simulink model "DoubleJoints_Algorithm"  (R2018b)
settings: Solver=FixedStepDiscrete  StartTime=0.0  StopTime=Inf  FixedStep=0.001  RelTol=1e-3  EnableMultiTasking=on
undefined symbols (not defined in the file): J2, J7, Motor_Current, Motor_Position, Motor_Velocity, Send_GUIdata
libraries: c280xlib x20, simulink x9, dspsrcs4 x2, idelinklib_common x1
(part 2 of 3)

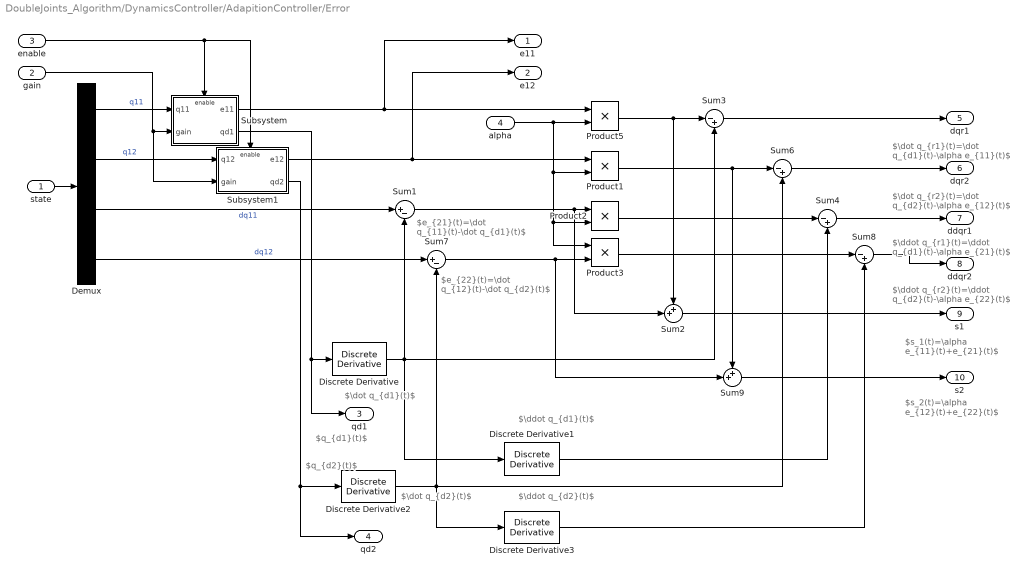
== system DoubleJoints_Algorithm/DynamicsController/AdapitionController/Error  ==
  note: $\dot q_{r2}(t)=\dot q_{d2}(t)-\alpha e_{12}(t)$
  note: $\dot q_{r1}(t)=\dot q_{d1}(t)-\alpha e_{11}(t)$
  note: $\ddot q_{r1}(t)=\ddot q_{d1}(t)-\alpha e_{21}(t)$
  note: $\ddot q_{r2}(t)=\ddot q_{d2}(t)-\alpha e_{22}(t)$
  note: $s_1(t)=\alpha e_{11}(t)+e_{21}(t)$
  note: $s_2(t)=\alpha e_{12}(t)+e_{22}(t)$
  note: $e_{21}(t)=\dot q_{11}(t)-\dot q_{d1}(t)$
  note: $e_{22}(t)=\dot q_{12}(t)-\dot q_{d2}(t)$
  note: $\dot q_{d2}(t)$
  note: $\dot q_{d1}(t)$
  note: $\ddot q_{d1}(t)$
  note: $q_{d1}(t)$
  note: $\ddot q_{d2}(t)$
  note: $q_{d2}(t)$
  state : Inport
  gain : Inport  Port=2
  enable : Inport  Port=3
  alpha : Inport  Port=4
  Demux : Demux
  Discrete Derivative{,1..3} (4 alike) : simulink/Discrete/Discrete Derivative  gainval=1.0  ICPrevScaledInput=0.0  OutMin=[]  OutMax=[]  OutDataType=fixdt(1, 16)  OutScaling=2^-10  DoSatur=off
  Product{1..3,5} (4 alike) : Product
  Subsystem : Subsystem  Priority=1
      settings: RTWSystemCode=Nonreusable function
  Subsystem1 : Subsystem  Priority=2
      settings: RTWSystemCode=Nonreusable function
  Sum1 : Sum  Inputs=|+-
  Sum2 : Sum  Inputs=++|
  Sum{3..4,6,8} (4 alike) : Sum  Inputs=|-+
  Sum7 : Sum  Inputs=|+-
  Sum9 : Sum  Inputs=++|
  e11 : Outport
  e12 : Outport  Port=2
  qd1 : Outport  Port=3
  qd2 : Outport  Port=4
  dqr1 : Outport  Port=5
  dqr2 : Outport  Port=6
  ddqr1 : Outport  Port=7
  ddqr2 : Outport  Port=8
  s1 : Outport  Port=9
  s2 : Outport  Port=10
  wires:
  state/1 -> Demux/1
  Demux/1 -> Subsystem/1(q11)  "q11"
  Demux/3 -> Sum1/1  "dq11"
  Subsystem/2(qd1) -> Discrete Derivative/1, qd1/1
  Product5/1 -> Sum3/1, Sum2/1
  Sum3/1 -> dqr1/1
  Sum1/1 -> Product2/1, Sum2/2
  Product2/1 -> Sum4/1
  Discrete Derivative/1 -> Sum3/2, Discrete Derivative1/1, Sum1/2
  Sum4/1 -> ddqr1/1
  Sum2/1 -> s1/1
  Demux/2 -> Subsystem1/1(q12)  "q12"
  Product1/1 -> Sum6/1, Sum9/1
  Sum6/1 -> dqr2/1
  Demux/4 -> Sum7/1  "dq12"
  Sum7/1 -> Sum9/2, Product3/2
  Product3/1 -> Sum8/1
  Subsystem1/2(qd2) -> qd2/1, Discrete Derivative2/1
  Sum8/1 -> ddqr2/1
  Sum9/1 -> s2/1
  alpha/1 -> Product5/2, Product1/2, Product2/2, Product3/1
  Discrete Derivative1/1 -> Sum4/2
  Discrete Derivative3/1 -> Sum8/2
  Discrete Derivative2/1 -> Discrete Derivative3/1, Sum6/2, Sum7/2
  enable/1 -> Subsystem/Enable, Subsystem1/Enable
  Subsystem/1(e11) -> e11/1, Product5/1
  Subsystem1/1(e12) -> e12/1, Product1/1
  gain/1 -> Subsystem1/2(gain), Subsystem/2(gain)

== system DoubleJoints_Algorithm/DynamicsController/DriverTwoMotor/BottomDriver ==
  SelectJoint1 : Inport
  SelectJoint2 : Inport  Port=2
  MSG1 : Inport  Port=3
  MSG2 : Inport  Port=4
  Enable : EnablePort
  Judgement : Subsystem
  Relational Operator : RelationalOperator  Operator=~=  OutDataTypeStr=boolean  RndMeth=Simplest
  wires:
  MSG1/1 -> Judgement/3(MSG1)
  MSG2/1 -> Judgement/4(MSG2)
  SelectJoint1/1 -> Judgement/1(SelectJointOne), Relational Operator/1
  SelectJoint2/1 -> Judgement/2(SelectJointTwo), Relational Operator/2
  Relational Operator/1 -> Judgement/Enable

== system DoubleJoints_Algorithm/DynamicsController/DriverTwoMotor/驱动器指令 ==
  Current1 : Inport
  Current2 : Inport  Port=2
  enable : Inport  Port=3
  Chart2 : Stateflow chart  TreatAsAtomicUnit=on
  Data Store Read : DataStoreRead  DataStoreName=StartRobot
  Data Type Conversion1 : DataTypeConversion  OutDataTypeStr=uint8
  Data Type Conversion2 : DataTypeConversion  OutDataTypeStr=uint16
  Data Type Conversion3 : DataTypeConversion  OutDataTypeStr=uint8
  Data Type Conversion4 : DataTypeConversion  OutDataTypeStr=uint16
  Data Type Conversion7 : DataTypeConversion  OutDataTypeStr=uint16
  MSG1 : Outport
  MSG2 : Outport  Port=2
  wires:
  Data Type Conversion1/1 -> MSG1/1
  Chart2/1(MSG1) -> Data Type Conversion1/1
  Current2/1 -> Data Type Conversion7/1
  Data Type Conversion7/1 -> Chart2/2(Current2)
  Current1/1 -> Data Type Conversion2/1
  Data Type Conversion2/1 -> Chart2/1(Current1)
  Data Type Conversion3/1 -> MSG2/1
  Chart2/2(MSG2) -> Data Type Conversion3/1
  Data Type Conversion4/1 -> Chart2/3(write)
  enable/1 -> Data Type Conversion4/1
  Data Store Read/1 -> Chart2/4(StartRobot)

== system DoubleJoints_Algorithm/DynamicsController/GetAngle1/Joint1 ==
  note: 内转子位置的脉冲值
  Action Port : ActionPort
  Data Store Read5 : DataStoreRead  DataStoreName=Motor_Position  DataStoreElements=Motor_Position(1)
  Joint1 : Outport
  wires:
  Data Store Read5/1 -> Joint1/1

== system DoubleJoints_Algorithm/DynamicsController/GetAngle1/Joint2 ==
  Action Port : ActionPort
  Data Store Read5 : DataStoreRead  DataStoreName=Motor_Position  DataStoreElements=Motor_Position(2)
  Joint2 : Outport
  wires:
  Data Store Read5/1 -> Joint2/1

== system DoubleJoints_Algorithm/DynamicsController/GetAngle1/Joint3 ==
  Action Port : ActionPort
  Data Store Read5 : DataStoreRead  DataStoreName=Motor_Position  DataStoreElements=Motor_Position(3)
  Joint3 : Outport
  wires:
  Data Store Read5/1 -> Joint3/1

== system DoubleJoints_Algorithm/DynamicsController/GetAngle1/Joint4 ==
  Action Port : ActionPort
  Data Store Read5 : DataStoreRead  DataStoreName=Motor_Position  DataStoreElements=Motor_Position(4)
  Joint4 : Outport
  wires:
  Data Store Read5/1 -> Joint4/1

== system DoubleJoints_Algorithm/DynamicsController/GetAngle1/Joint5 ==
  Action Port : ActionPort
  Data Store Read5 : DataStoreRead  DataStoreName=Motor_Position  DataStoreElements=Motor_Position(5)
  Joint5 : Outport
  wires:
  Data Store Read5/1 -> Joint5/1

== system DoubleJoints_Algorithm/DynamicsController/GetAngle1/Joint6 ==
  Action Port : ActionPort
  Data Store Read5 : DataStoreRead  DataStoreName=Motor_Position  DataStoreElements=Motor_Position(6)
  Joint6 : Outport
  wires:
  Data Store Read5/1 -> Joint6/1

== system DoubleJoints_Algorithm/DynamicsController/GetAngle2/Joint1 ==
  note: 内转子位置的脉冲值
  Action Port : ActionPort
  Data Store Read5 : DataStoreRead  DataStoreName=Motor_Position  DataStoreElements=Motor_Position(1)
  Joint1 : Outport
  wires:
  Data Store Read5/1 -> Joint1/1

== system DoubleJoints_Algorithm/DynamicsController/GetAngle2/Joint2 ==
  Action Port : ActionPort
  Data Store Read5 : DataStoreRead  DataStoreName=Motor_Position  DataStoreElements=Motor_Position(2)
  Joint2 : Outport
  wires:
  Data Store Read5/1 -> Joint2/1

== system DoubleJoints_Algorithm/DynamicsController/GetAngle2/Joint3 ==
  Action Port : ActionPort
  Data Store Read5 : DataStoreRead  DataStoreName=Motor_Position  DataStoreElements=Motor_Position(3)
  Joint3 : Outport
  wires:
  Data Store Read5/1 -> Joint3/1

== system DoubleJoints_Algorithm/DynamicsController/GetAngle2/Joint4 ==
  Action Port : ActionPort
  Data Store Read5 : DataStoreRead  DataStoreName=Motor_Position  DataStoreElements=Motor_Position(4)
  Joint4 : Outport
  wires:
  Data Store Read5/1 -> Joint4/1

== system DoubleJoints_Algorithm/DynamicsController/GetAngle2/Joint5 ==
  Action Port : ActionPort
  Data Store Read5 : DataStoreRead  DataStoreName=Motor_Position  DataStoreElements=Motor_Position(5)
  Joint5 : Outport
  wires:
  Data Store Read5/1 -> Joint5/1

== system DoubleJoints_Algorithm/DynamicsController/GetAngle2/Joint6 ==
  Action Port : ActionPort
  Data Store Read5 : DataStoreRead  DataStoreName=Motor_Position  DataStoreElements=Motor_Position(6)
  Joint6 : Outport
  wires:
  Data Store Read5/1 -> Joint6/1

== system DoubleJoints_Algorithm/DynamicsController/GetAngleSpeed/Joint1 ==
  note: 内转子速度
      | 的脉冲值
  Action Port : ActionPort  ActionType=case
  Data Store Read1 : DataStoreRead  DataStoreName=Motor_Velocity  DataStoreElements=Motor_Velocity(1)
  Joint1_Velocity : Outport
  wires:
  Data Store Read1/1 -> Joint1_Velocity/1

== system DoubleJoints_Algorithm/DynamicsController/GetAngleSpeed/Joint2 ==
  note: 内转子速度
      | 的脉冲值
  Action Port : ActionPort  ActionType=case
  Data Store Read1 : DataStoreRead  DataStoreName=Motor_Velocity  DataStoreElements=Motor_Velocity(2)
  Joint2_Velocity : Outport
  wires:
  Data Store Read1/1 -> Joint2_Velocity/1

== system DoubleJoints_Algorithm/DynamicsController/GetAngleSpeed/Joint3 ==
  note: 内转子速度
      | 的脉冲值
  Action Port : ActionPort  ActionType=case
  Data Store Read1 : DataStoreRead  DataStoreName=Motor_Velocity  DataStoreElements=Motor_Velocity(3)
  Joint3_Velocity : Outport
  wires:
  Data Store Read1/1 -> Joint3_Velocity/1

== system DoubleJoints_Algorithm/DynamicsController/GetAngleSpeed/Joint4 ==
  note: 内转子速度
      | 的脉冲值
  Action Port : ActionPort  ActionType=case
  Data Store Read1 : DataStoreRead  DataStoreName=Motor_Velocity  DataStoreElements=Motor_Velocity(4)
  Joint4_Velocity : Outport
  wires:
  Data Store Read1/1 -> Joint4_Velocity/1

== system DoubleJoints_Algorithm/DynamicsController/GetAngleSpeed/Joint5 ==
  note: 内转子速度
      | 的脉冲值
  Action Port : ActionPort  ActionType=case
  Data Store Read1 : DataStoreRead  DataStoreName=Motor_Velocity  DataStoreElements=Motor_Velocity(5)
  Joint5_Velocity : Outport
  wires:
  Data Store Read1/1 -> Joint5_Velocity/1

== system DoubleJoints_Algorithm/DynamicsController/GetAngleSpeed/Joint6 ==
  note: 内转子速度
      | 的脉冲值
  Action Port : ActionPort  ActionType=case
  Data Store Read1 : DataStoreRead  DataStoreName=Motor_Velocity  DataStoreElements=Motor_Velocity(6)
  Joint6_Velocity : Outport
  wires:
  Data Store Read1/1 -> Joint6_Velocity/1

== system DoubleJoints_Algorithm/DynamicsController/GetAngleSpeed1/Joint1 ==
  note: 内转子速度
      | 的脉冲值
  Action Port : ActionPort  ActionType=case
  Data Store Read1 : DataStoreRead  DataStoreName=Motor_Velocity  DataStoreElements=Motor_Velocity(1)
  Joint1_Velocity : Outport
  wires:
  Data Store Read1/1 -> Joint1_Velocity/1

== system DoubleJoints_Algorithm/DynamicsController/GetAngleSpeed1/Joint2 ==
  note: 内转子速度
      | 的脉冲值
  Action Port : ActionPort  ActionType=case
  Data Store Read1 : DataStoreRead  DataStoreName=Motor_Velocity  DataStoreElements=Motor_Velocity(2)
  Joint2_Velocity : Outport
  wires:
  Data Store Read1/1 -> Joint2_Velocity/1

== system DoubleJoints_Algorithm/DynamicsController/GetAngleSpeed1/Joint3 ==
  note: 内转子速度
      | 的脉冲值
  Action Port : ActionPort  ActionType=case
  Data Store Read1 : DataStoreRead  DataStoreName=Motor_Velocity  DataStoreElements=Motor_Velocity(3)
  Joint3_Velocity : Outport
  wires:
  Data Store Read1/1 -> Joint3_Velocity/1

== system DoubleJoints_Algorithm/DynamicsController/GetAngleSpeed1/Joint4 ==
  note: 内转子速度
      | 的脉冲值
  Action Port : ActionPort  ActionType=case
  Data Store Read1 : DataStoreRead  DataStoreName=Motor_Velocity  DataStoreElements=Motor_Velocity(4)
  Joint4_Velocity : Outport
  wires:
  Data Store Read1/1 -> Joint4_Velocity/1

== system DoubleJoints_Algorithm/DynamicsController/GetAngleSpeed1/Joint5 ==
  note: 内转子速度
      | 的脉冲值
  Action Port : ActionPort  ActionType=case
  Data Store Read1 : DataStoreRead  DataStoreName=Motor_Velocity  DataStoreElements=Motor_Velocity(5)
  Joint5_Velocity : Outport
  wires:
  Data Store Read1/1 -> Joint5_Velocity/1

== system DoubleJoints_Algorithm/DynamicsController/GetAngleSpeed1/Joint6 ==
  note: 内转子速度
      | 的脉冲值
  Action Port : ActionPort  ActionType=case
  Data Store Read1 : DataStoreRead  DataStoreName=Motor_Velocity  DataStoreElements=Motor_Velocity(6)
  Joint6_Velocity : Outport
  wires:
  Data Store Read1/1 -> Joint6_Velocity/1

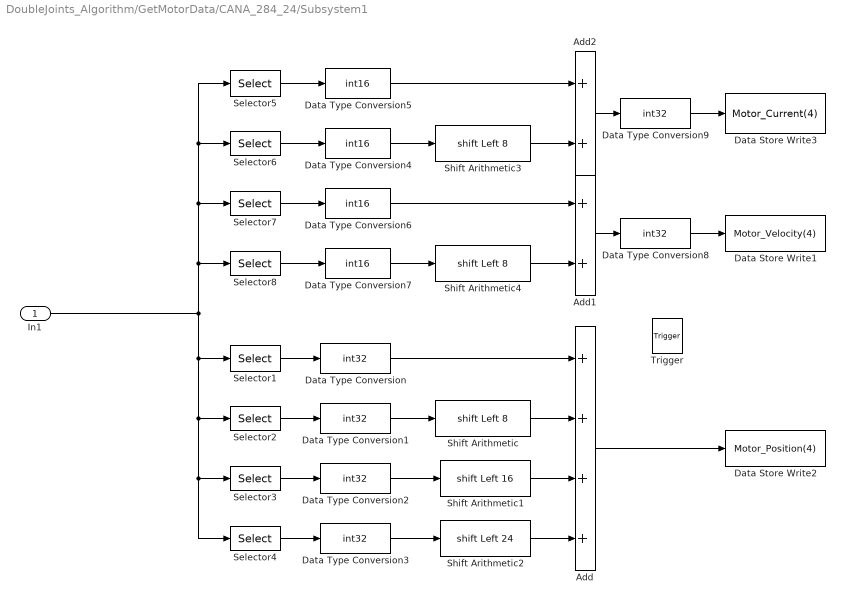
== system DoubleJoints_Algorithm/GetMotorData/CANA_284_24/Subsystem1 ==
  In1 : Inport
  Trigger : TriggerPort  TriggerType=function-call  VariantControl=Variant  PortDimensions=1
  Add : Sum  Inputs=4
  Add1 : Sum  Inputs=2
  Add2 : Sum  Inputs=2
  Data Store Write1 : DataStoreWrite  DataStoreName=Motor_Velocity  DataStoreElements=Motor_Velocity(4)
  Data Store Write2 : DataStoreWrite  DataStoreName=Motor_Position  DataStoreElements=Motor_Position(4)
  Data Store Write3 : DataStoreWrite  DataStoreName=Motor_Current  DataStoreElements=Motor_Current(4)
  Data Type Conversion{,1..3,8..9} (6 alike) : DataTypeConversion  OutDataTypeStr=int32
  Data Type Conversion{4..7} (4 alike) : DataTypeConversion  OutDataTypeStr=int16
  Selector1 : Selector  IndexMode=Zero-based  InputPortWidth=8  IndexOptions=Index vector (dialog)  Indices=4  OutputSizes=1
  Selector2 : Selector  IndexMode=Zero-based  InputPortWidth=8  IndexOptions=Index vector (dialog)  Indices=5  OutputSizes=1
  Selector3 : Selector  IndexMode=Zero-based  InputPortWidth=8  IndexOptions=Index vector (dialog)  Indices=6  OutputSizes=1
  Selector4 : Selector  IndexMode=Zero-based  InputPortWidth=8  IndexOptions=Index vector (dialog)  Indices=7  OutputSizes=1
  Selector5 : Selector  IndexMode=Zero-based  InputPortWidth=8  IndexOptions=Index vector (dialog)  Indices=0  OutputSizes=1
  Selector6 : Selector  IndexMode=Zero-based  InputPortWidth=8  IndexOptions=Index vector (dialog)  Indices=1  OutputSizes=1
  Selector7 : Selector  IndexMode=Zero-based  InputPortWidth=8  IndexOptions=Index vector (dialog)  Indices=2  OutputSizes=1
  Selector8 : Selector  IndexMode=Zero-based  InputPortWidth=8  IndexOptions=Index vector (dialog)  Indices=3  OutputSizes=1
  Shift Arithmetic : ArithShift  BitShiftNumber=8  BitShiftDirection=Left
  Shift Arithmetic1 : ArithShift  BitShiftNumber=16  BitShiftDirection=Left
  Shift Arithmetic2 : ArithShift  BitShiftNumber=24  BitShiftDirection=Left
  Shift Arithmetic3 : ArithShift  BitShiftNumber=8  BitShiftDirection=Left
  Shift Arithmetic4 : ArithShift  BitShiftNumber=8  BitShiftDirection=Left
  wires:
  Selector3/1 -> Data Type Conversion2/1
  Shift Arithmetic/1 -> Add/2
  Shift Arithmetic2/1 -> Add/4
  Data Type Conversion/1 -> Add/1
  Selector1/1 -> Data Type Conversion/1
  Selector4/1 -> Data Type Conversion3/1
  Add/1 -> Data Store Write2/1
  Shift Arithmetic1/1 -> Add/3
  Selector2/1 -> Data Type Conversion1/1
  Data Type Conversion7/1 -> Shift Arithmetic4/1
  Data Type Conversion6/1 -> Add1/1
  Selector7/1 -> Data Type Conversion6/1
  Selector8/1 -> Data Type Conversion7/1
  Selector6/1 -> Data Type Conversion4/1
  In1/1 -> Selector3/1, Selector4/1, Selector2/1, Selector1/1, Selector5/1, Selector6/1, Selector7/1, Selector8/1
  Add1/1 -> Data Type Conversion8/1
  Shift Arithmetic4/1 -> Add1/2
  Data Type Conversion1/1 -> Shift Arithmetic/1
  Data Type Conversion2/1 -> Shift Arithmetic1/1
  Data Type Conversion3/1 -> Shift Arithmetic2/1
  Selector5/1 -> Data Type Conversion5/1
  Data Type Conversion4/1 -> Shift Arithmetic3/1
  Data Type Conversion8/1 -> Data Store Write1/1
  Shift Arithmetic3/1 -> Add2/2
  Data Type Conversion5/1 -> Add2/1
  Add2/1 -> Data Type Conversion9/1
  Data Type Conversion9/1 -> Data Store Write3/1

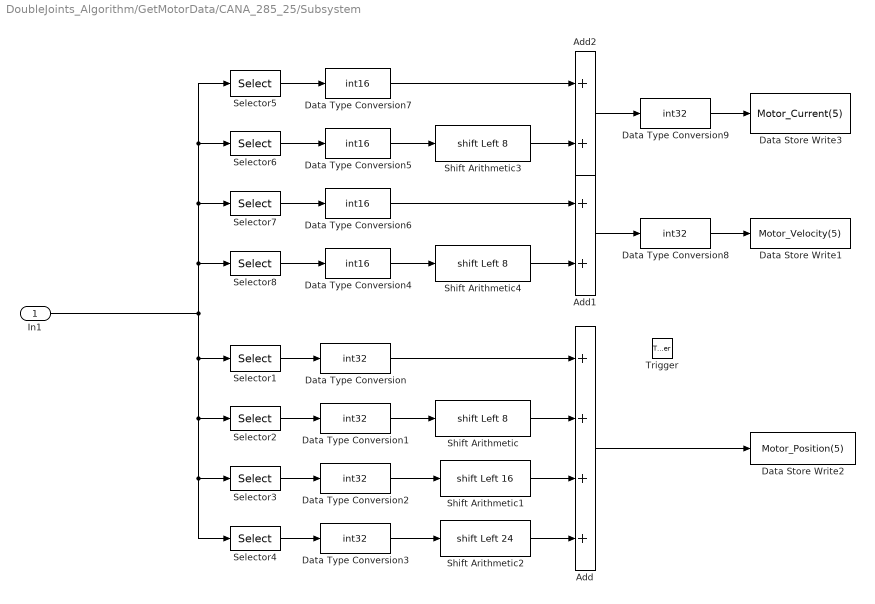
== system DoubleJoints_Algorithm/GetMotorData/CANA_285_25/Subsystem ==
  In1 : Inport
  Trigger : TriggerPort  TriggerType=function-call  VariantControl=Variant  PortDimensions=1
  Add : Sum  Inputs=4
  Add1 : Sum  Inputs=2
  Add2 : Sum  Inputs=2
  Data Store Write1 : DataStoreWrite  DataStoreName=Motor_Velocity  DataStoreElements=Motor_Velocity(5)
  Data Store Write2 : DataStoreWrite  DataStoreName=Motor_Position  DataStoreElements=Motor_Position(5)
  Data Store Write3 : DataStoreWrite  DataStoreName=Motor_Current  DataStoreElements=Motor_Current(5)
  Data Type Conversion{,1..3,8..9} (6 alike) : DataTypeConversion  OutDataTypeStr=int32
  Data Type Conversion{4..7} (4 alike) : DataTypeConversion  OutDataTypeStr=int16
  Selector1 : Selector  IndexMode=Zero-based  InputPortWidth=8  IndexOptions=Index vector (dialog)  Indices=4  OutputSizes=1
  Selector2 : Selector  IndexMode=Zero-based  InputPortWidth=8  IndexOptions=Index vector (dialog)  Indices=5  OutputSizes=1
  Selector3 : Selector  IndexMode=Zero-based  InputPortWidth=8  IndexOptions=Index vector (dialog)  Indices=6  OutputSizes=1
  Selector4 : Selector  IndexMode=Zero-based  InputPortWidth=8  IndexOptions=Index vector (dialog)  Indices=7  OutputSizes=1
  Selector5 : Selector  IndexMode=Zero-based  InputPortWidth=8  IndexOptions=Index vector (dialog)  Indices=0  OutputSizes=1
  Selector6 : Selector  IndexMode=Zero-based  InputPortWidth=8  IndexOptions=Index vector (dialog)  Indices=1  OutputSizes=1
  Selector7 : Selector  IndexMode=Zero-based  InputPortWidth=8  IndexOptions=Index vector (dialog)  Indices=2  OutputSizes=1
  Selector8 : Selector  IndexMode=Zero-based  InputPortWidth=8  IndexOptions=Index vector (dialog)  Indices=3  OutputSizes=1
  Shift Arithmetic : ArithShift  BitShiftNumber=8  BitShiftDirection=Left
  Shift Arithmetic1 : ArithShift  BitShiftNumber=16  BitShiftDirection=Left
  Shift Arithmetic2 : ArithShift  BitShiftNumber=24  BitShiftDirection=Left
  Shift Arithmetic3 : ArithShift  BitShiftNumber=8  BitShiftDirection=Left
  Shift Arithmetic4 : ArithShift  BitShiftNumber=8  BitShiftDirection=Left
  wires:
  Selector3/1 -> Data Type Conversion2/1
  Shift Arithmetic/1 -> Add/2
  Shift Arithmetic2/1 -> Add/4
  Data Type Conversion/1 -> Add/1
  Selector1/1 -> Data Type Conversion/1
  Selector4/1 -> Data Type Conversion3/1
  Add/1 -> Data Store Write2/1
  Shift Arithmetic1/1 -> Add/3
  Selector2/1 -> Data Type Conversion1/1
  Selector5/1 -> Data Type Conversion7/1
  Selector8/1 -> Data Type Conversion4/1
  Data Type Conversion4/1 -> Shift Arithmetic4/1
  Data Type Conversion6/1 -> Add1/1
  Selector7/1 -> Data Type Conversion6/1
  Selector6/1 -> Data Type Conversion5/1
  In1/1 -> Selector3/1, Selector4/1, Selector2/1, Selector1/1, Selector5/1, Selector6/1, Selector7/1, Selector8/1
  Add1/1 -> Data Type Conversion8/1
  Data Type Conversion1/1 -> Shift Arithmetic/1
  Data Type Conversion2/1 -> Shift Arithmetic1/1
  Data Type Conversion3/1 -> Shift Arithmetic2/1
  Data Type Conversion5/1 -> Shift Arithmetic3/1
  Shift Arithmetic4/1 -> Add1/2
  Shift Arithmetic3/1 -> Add2/2
  Data Type Conversion7/1 -> Add2/1
  Add2/1 -> Data Type Conversion9/1
  Data Type Conversion8/1 -> Data Store Write1/1
  Data Type Conversion9/1 -> Data Store Write3/1

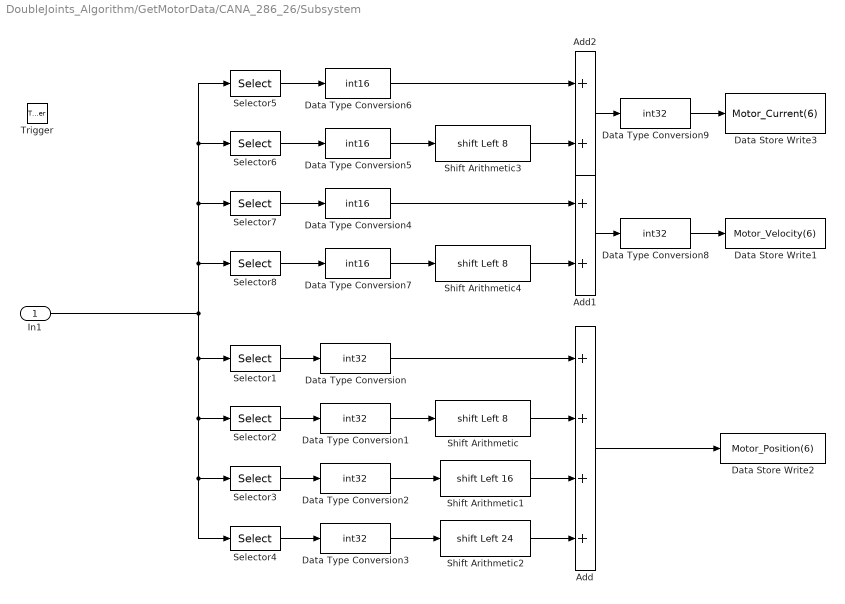
== system DoubleJoints_Algorithm/GetMotorData/CANA_286_26/Subsystem ==
  In1 : Inport
  Trigger : TriggerPort  TriggerType=function-call  VariantControl=Variant  PortDimensions=1
  Add : Sum  Inputs=4
  Add1 : Sum  Inputs=2
  Add2 : Sum  Inputs=2
  Data Store Write1 : DataStoreWrite  DataStoreName=Motor_Velocity  DataStoreElements=Motor_Velocity(6)
  Data Store Write2 : DataStoreWrite  DataStoreName=Motor_Position  DataStoreElements=Motor_Position(6)
  Data Store Write3 : DataStoreWrite  DataStoreName=Motor_Current  DataStoreElements=Motor_Current(6)
  Data Type Conversion{,1..3,8..9} (6 alike) : DataTypeConversion  OutDataTypeStr=int32
  Data Type Conversion{4..7} (4 alike) : DataTypeConversion  OutDataTypeStr=int16
  Selector1 : Selector  IndexMode=Zero-based  InputPortWidth=8  IndexOptions=Index vector (dialog)  Indices=4  OutputSizes=1
  Selector2 : Selector  IndexMode=Zero-based  InputPortWidth=8  IndexOptions=Index vector (dialog)  Indices=5  OutputSizes=1
  Selector3 : Selector  IndexMode=Zero-based  InputPortWidth=8  IndexOptions=Index vector (dialog)  Indices=6  OutputSizes=1
  Selector4 : Selector  IndexMode=Zero-based  InputPortWidth=8  IndexOptions=Index vector (dialog)  Indices=7  OutputSizes=1
  Selector5 : Selector  IndexMode=Zero-based  InputPortWidth=8  IndexOptions=Index vector (dialog)  Indices=0  OutputSizes=1
  Selector6 : Selector  IndexMode=Zero-based  InputPortWidth=8  IndexOptions=Index vector (dialog)  Indices=1  OutputSizes=1
  Selector7 : Selector  IndexMode=Zero-based  InputPortWidth=8  IndexOptions=Index vector (dialog)  Indices=2  OutputSizes=1
  Selector8 : Selector  IndexMode=Zero-based  InputPortWidth=8  IndexOptions=Index vector (dialog)  Indices=3  OutputSizes=1
  Shift Arithmetic : ArithShift  BitShiftNumber=8  BitShiftDirection=Left
  Shift Arithmetic1 : ArithShift  BitShiftNumber=16  BitShiftDirection=Left
  Shift Arithmetic2 : ArithShift  BitShiftNumber=24  BitShiftDirection=Left
  Shift Arithmetic3 : ArithShift  BitShiftNumber=8  BitShiftDirection=Left
  Shift Arithmetic4 : ArithShift  BitShiftNumber=8  BitShiftDirection=Left
  wires:
  Selector3/1 -> Data Type Conversion2/1
  Shift Arithmetic/1 -> Add/2
  Shift Arithmetic2/1 -> Add/4
  Data Type Conversion/1 -> Add/1
  Selector1/1 -> Data Type Conversion/1
  Selector4/1 -> Data Type Conversion3/1
  Add/1 -> Data Store Write2/1
  Shift Arithmetic1/1 -> Add/3
  Selector2/1 -> Data Type Conversion1/1
  Selector5/1 -> Data Type Conversion6/1
  Data Type Conversion7/1 -> Shift Arithmetic4/1
  Selector7/1 -> Data Type Conversion4/1
  Selector8/1 -> Data Type Conversion7/1
  Selector6/1 -> Data Type Conversion5/1
  In1/1 -> Selector3/1, Selector4/1, Selector2/1, Selector1/1, Selector5/1, Selector6/1, Selector7/1, Selector8/1
  Add1/1 -> Data Type Conversion8/1
  Data Type Conversion1/1 -> Shift Arithmetic/1
  Data Type Conversion2/1 -> Shift Arithmetic1/1
  Data Type Conversion3/1 -> Shift Arithmetic2/1
  Shift Arithmetic4/1 -> Add1/2
  Data Type Conversion4/1 -> Add1/1
  Data Type Conversion5/1 -> Shift Arithmetic3/1
  Data Type Conversion6/1 -> Add2/1
  Shift Arithmetic3/1 -> Add2/2
  Add2/1 -> Data Type Conversion9/1
  Data Type Conversion8/1 -> Data Store Write1/1
  Data Type Conversion9/1 -> Data Store Write3/1

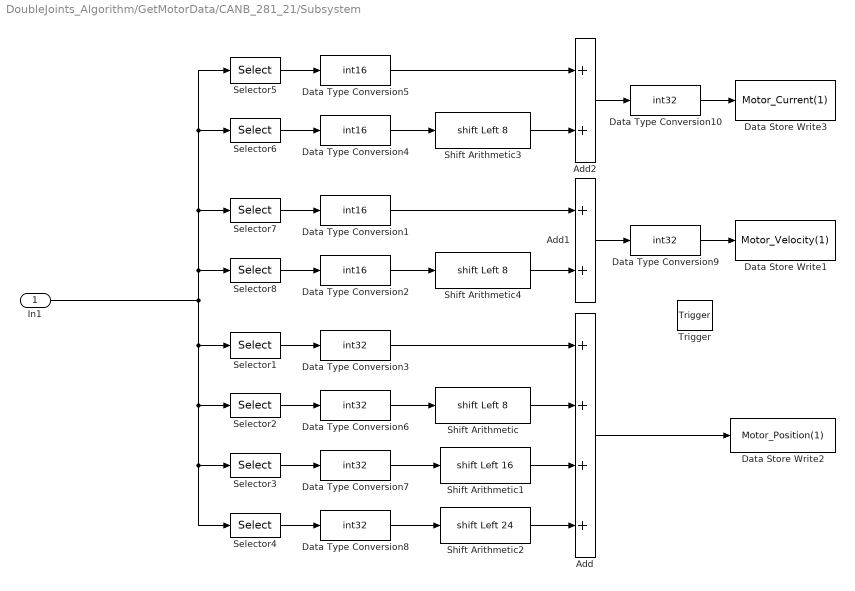
== system DoubleJoints_Algorithm/GetMotorData/CANB_281_21/Subsystem ==
  In1 : Inport
  Trigger : TriggerPort  TriggerType=function-call  VariantControl=Variant  PortDimensions=1
  Add : Sum  Inputs=4
  Add1 : Sum  Inputs=2
  Add2 : Sum  Inputs=2
  Data Store Write1 : DataStoreWrite  DataStoreName=Motor_Velocity  DataStoreElements=Motor_Velocity(1)
  Data Store Write2 : DataStoreWrite  DataStoreName=Motor_Position  DataStoreElements=Motor_Position(1)
  Data Store Write3 : DataStoreWrite  DataStoreName=Motor_Current  DataStoreElements=Motor_Current(1)
  Data Type Conversion{1..2,4..5} (4 alike) : DataTypeConversion  OutDataTypeStr=int16
  Data Type Conversion{3,6..10} (6 alike) : DataTypeConversion  OutDataTypeStr=int32
  Selector1 : Selector  IndexMode=Zero-based  InputPortWidth=8  IndexOptions=Index vector (dialog)  Indices=4  OutputSizes=1
  Selector2 : Selector  IndexMode=Zero-based  InputPortWidth=8  IndexOptions=Index vector (dialog)  Indices=5  OutputSizes=1
  Selector3 : Selector  IndexMode=Zero-based  InputPortWidth=8  IndexOptions=Index vector (dialog)  Indices=6  OutputSizes=1
  Selector4 : Selector  IndexMode=Zero-based  InputPortWidth=8  IndexOptions=Index vector (dialog)  Indices=7  OutputSizes=1
  Selector5 : Selector  IndexMode=Zero-based  InputPortWidth=8  IndexOptions=Index vector (dialog)  Indices=0  OutputSizes=1
  Selector6 : Selector  IndexMode=Zero-based  InputPortWidth=8  IndexOptions=Index vector (dialog)  Indices=1  OutputSizes=1
  Selector7 : Selector  IndexMode=Zero-based  InputPortWidth=8  IndexOptions=Index vector (dialog)  Indices=2  OutputSizes=1
  Selector8 : Selector  IndexMode=Zero-based  InputPortWidth=8  IndexOptions=Index vector (dialog)  Indices=3  OutputSizes=1
  Shift Arithmetic : ArithShift  BitShiftNumber=8  BitShiftDirection=Left
  Shift Arithmetic1 : ArithShift  BitShiftNumber=16  BitShiftDirection=Left
  Shift Arithmetic2 : ArithShift  BitShiftNumber=24  BitShiftDirection=Left
  Shift Arithmetic3 : ArithShift  BitShiftNumber=8  BitShiftDirection=Left
  Shift Arithmetic4 : ArithShift  BitShiftNumber=8  BitShiftDirection=Left
  wires:
  Data Type Conversion7/1 -> Shift Arithmetic1/1
  Shift Arithmetic/1 -> Add/2
  Selector2/1 -> Data Type Conversion6/1
  Selector3/1 -> Data Type Conversion7/1
  Shift Arithmetic2/1 -> Add/4
  Data Type Conversion3/1 -> Add/1
  Selector1/1 -> Data Type Conversion3/1
  Data Type Conversion8/1 -> Shift Arithmetic2/1
  Add/1 -> Data Store Write2/1
  Selector4/1 -> Data Type Conversion8/1
  Shift Arithmetic1/1 -> Add/3
  Data Type Conversion6/1 -> Shift Arithmetic/1
  Data Type Conversion2/1 -> Shift Arithmetic4/1
  Shift Arithmetic4/1 -> Add1/2
  Data Type Conversion1/1 -> Add1/1
  Selector7/1 -> Data Type Conversion1/1
  Selector8/1 -> Data Type Conversion2/1
  Selector6/1 -> Data Type Conversion4/1
  In1/1 -> Selector3/1, Selector4/1, Selector2/1, Selector1/1, Selector5/1, Selector6/1, Selector7/1, Selector8/1
  Add1/1 -> Data Type Conversion9/1
  Selector5/1 -> Data Type Conversion5/1
  Data Type Conversion4/1 -> Shift Arithmetic3/1
  Data Type Conversion9/1 -> Data Store Write1/1
  Shift Arithmetic3/1 -> Add2/2
  Data Type Conversion5/1 -> Add2/1
  Add2/1 -> Data Type Conversion10/1
  Data Type Conversion10/1 -> Data Store Write3/1

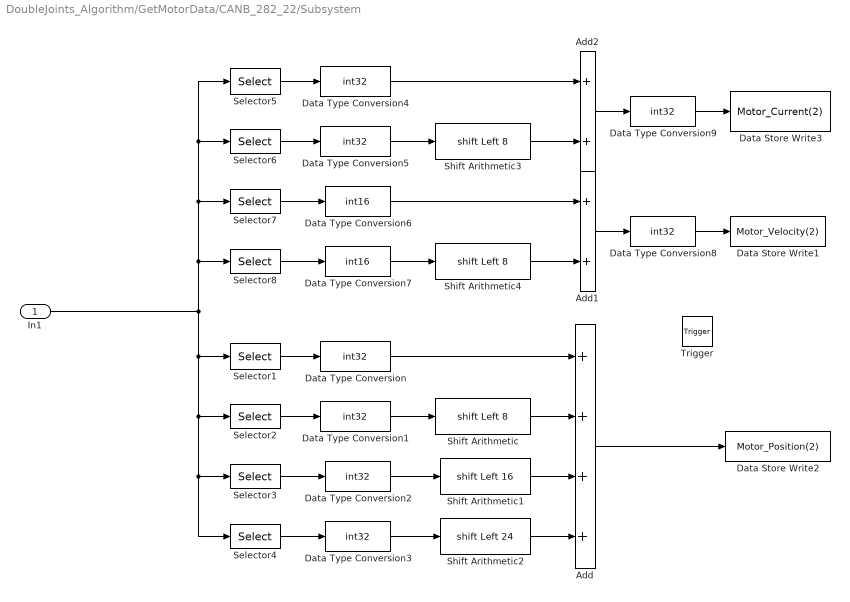
== system DoubleJoints_Algorithm/GetMotorData/CANB_282_22/Subsystem ==
  In1 : Inport
  Trigger : TriggerPort  TriggerType=function-call  VariantControl=Variant  PortDimensions=1
  Add : Sum  Inputs=4
  Add1 : Sum  Inputs=2
  Add2 : Sum  Inputs=2
  Data Store Write1 : DataStoreWrite  DataStoreName=Motor_Velocity  DataStoreElements=Motor_Velocity(2)
  Data Store Write2 : DataStoreWrite  DataStoreName=Motor_Position  DataStoreElements=Motor_Position(2)
  Data Store Write3 : DataStoreWrite  DataStoreName=Motor_Current  DataStoreElements=Motor_Current(2)
  Data Type Conversion{,1..5,8..9} (8 alike) : DataTypeConversion  OutDataTypeStr=int32
  Data Type Conversion6 : DataTypeConversion  OutDataTypeStr=int16
  Data Type Conversion7 : DataTypeConversion  OutDataTypeStr=int16
  Selector1 : Selector  IndexMode=Zero-based  InputPortWidth=8  IndexOptions=Index vector (dialog)  Indices=4  OutputSizes=1
  Selector2 : Selector  IndexMode=Zero-based  InputPortWidth=8  IndexOptions=Index vector (dialog)  Indices=5  OutputSizes=1
  Selector3 : Selector  IndexMode=Zero-based  InputPortWidth=8  IndexOptions=Index vector (dialog)  Indices=6  OutputSizes=1
  Selector4 : Selector  IndexMode=Zero-based  InputPortWidth=8  IndexOptions=Index vector (dialog)  Indices=7  OutputSizes=1
  Selector5 : Selector  IndexMode=Zero-based  InputPortWidth=8  IndexOptions=Index vector (dialog)  Indices=0  OutputSizes=1
  Selector6 : Selector  IndexMode=Zero-based  InputPortWidth=8  IndexOptions=Index vector (dialog)  Indices=1  OutputSizes=1
  Selector7 : Selector  IndexMode=Zero-based  InputPortWidth=8  IndexOptions=Index vector (dialog)  Indices=2  OutputSizes=1
  Selector8 : Selector  IndexMode=Zero-based  InputPortWidth=8  IndexOptions=Index vector (dialog)  Indices=3  OutputSizes=1
  Shift Arithmetic : ArithShift  BitShiftNumber=8  BitShiftDirection=Left
  Shift Arithmetic1 : ArithShift  BitShiftNumber=16  BitShiftDirection=Left
  Shift Arithmetic2 : ArithShift  BitShiftNumber=24  BitShiftDirection=Left
  Shift Arithmetic3 : ArithShift  BitShiftNumber=8  BitShiftDirection=Left
  Shift Arithmetic4 : ArithShift  BitShiftNumber=8  BitShiftDirection=Left
  wires:
  Data Type Conversion2/1 -> Shift Arithmetic1/1
  Shift Arithmetic/1 -> Add/2
  Selector2/1 -> Data Type Conversion1/1
  Selector3/1 -> Data Type Conversion2/1
  Shift Arithmetic2/1 -> Add/4
  Data Type Conversion/1 -> Add/1
  Selector1/1 -> Data Type Conversion/1
  Data Type Conversion3/1 -> Shift Arithmetic2/1
  Add/1 -> Data Store Write2/1
  Selector4/1 -> Data Type Conversion3/1
  Shift Arithmetic1/1 -> Add/3
  Data Type Conversion1/1 -> Shift Arithmetic/1
  In1/1 -> Selector3/1, Selector4/1, Selector2/1, Selector1/1, Selector8/1, Selector7/1, Selector6/1, Selector5/1
  Shift Arithmetic4/1 -> Add1/2
  Add1/1 -> Data Type Conversion8/1
  Data Type Conversion5/1 -> Shift Arithmetic3/1
  Selector8/1 -> Data Type Conversion7/1
  Data Type Conversion6/1 -> Add1/1
  Selector6/1 -> Data Type Conversion5/1
  Data Type Conversion7/1 -> Shift Arithmetic4/1
  Selector5/1 -> Data Type Conversion4/1
  Selector7/1 -> Data Type Conversion6/1
  Data Type Conversion8/1 -> Data Store Write1/1
  Shift Arithmetic3/1 -> Add2/2
  Data Type Conversion4/1 -> Add2/1
  Add2/1 -> Data Type Conversion9/1
  Data Type Conversion9/1 -> Data Store Write3/1

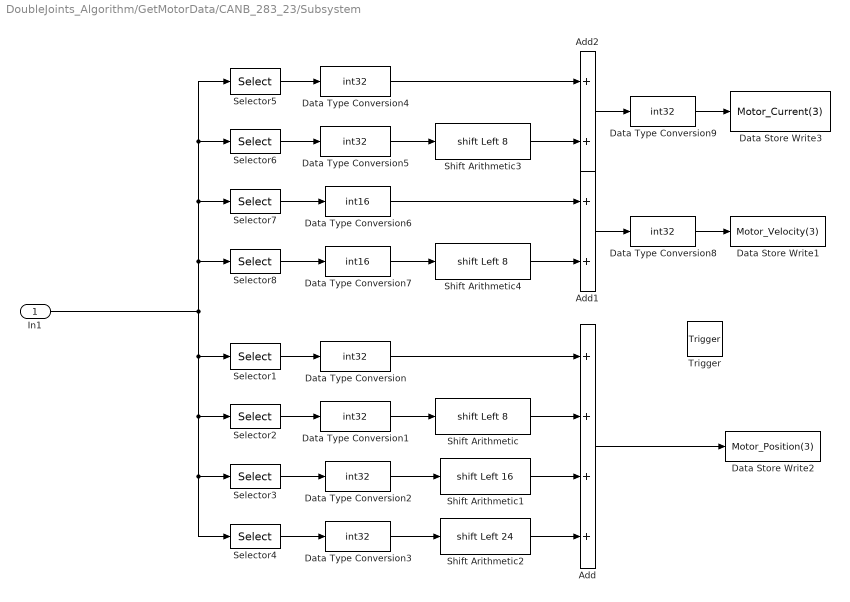
== system DoubleJoints_Algorithm/GetMotorData/CANB_283_23/Subsystem ==
  In1 : Inport
  Trigger : TriggerPort  TriggerType=function-call  VariantControl=Variant  PortDimensions=1
  Add : Sum  Inputs=4
  Add1 : Sum  Inputs=2
  Add2 : Sum  Inputs=2
  Data Store Write1 : DataStoreWrite  DataStoreName=Motor_Velocity  DataStoreElements=Motor_Velocity(3)
  Data Store Write2 : DataStoreWrite  DataStoreName=Motor_Position  DataStoreElements=Motor_Position(3)
  Data Store Write3 : DataStoreWrite  DataStoreName=Motor_Current  DataStoreElements=Motor_Current(3)
  Data Type Conversion{,1..5,8..9} (8 alike) : DataTypeConversion  OutDataTypeStr=int32
  Data Type Conversion6 : DataTypeConversion  OutDataTypeStr=int16
  Data Type Conversion7 : DataTypeConversion  OutDataTypeStr=int16
  Selector1 : Selector  IndexMode=Zero-based  InputPortWidth=8  IndexOptions=Index vector (dialog)  Indices=4  OutputSizes=1
  Selector2 : Selector  IndexMode=Zero-based  InputPortWidth=8  IndexOptions=Index vector (dialog)  Indices=5  OutputSizes=1
  Selector3 : Selector  IndexMode=Zero-based  InputPortWidth=8  IndexOptions=Index vector (dialog)  Indices=6  OutputSizes=1
  Selector4 : Selector  IndexMode=Zero-based  InputPortWidth=8  IndexOptions=Index vector (dialog)  Indices=7  OutputSizes=1
  Selector5 : Selector  IndexMode=Zero-based  InputPortWidth=8  IndexOptions=Index vector (dialog)  Indices=0  OutputSizes=1
  Selector6 : Selector  IndexMode=Zero-based  InputPortWidth=8  IndexOptions=Index vector (dialog)  Indices=1  OutputSizes=1
  Selector7 : Selector  IndexMode=Zero-based  InputPortWidth=8  IndexOptions=Index vector (dialog)  Indices=2  OutputSizes=1
  Selector8 : Selector  IndexMode=Zero-based  InputPortWidth=8  IndexOptions=Index vector (dialog)  Indices=3  OutputSizes=1
  Shift Arithmetic : ArithShift  BitShiftNumber=8  BitShiftDirection=Left
  Shift Arithmetic1 : ArithShift  BitShiftNumber=16  BitShiftDirection=Left
  Shift Arithmetic2 : ArithShift  BitShiftNumber=24  BitShiftDirection=Left
  Shift Arithmetic3 : ArithShift  BitShiftNumber=8  BitShiftDirection=Left
  Shift Arithmetic4 : ArithShift  BitShiftNumber=8  BitShiftDirection=Left
  wires:
  Data Type Conversion2/1 -> Shift Arithmetic1/1
  Shift Arithmetic/1 -> Add/2
  Selector2/1 -> Data Type Conversion1/1
  Selector3/1 -> Data Type Conversion2/1
  Shift Arithmetic2/1 -> Add/4
  Data Type Conversion/1 -> Add/1
  Selector1/1 -> Data Type Conversion/1
  Data Type Conversion3/1 -> Shift Arithmetic2/1
  Add/1 -> Data Store Write2/1
  Selector4/1 -> Data Type Conversion3/1
  Shift Arithmetic1/1 -> Add/3
  Data Type Conversion1/1 -> Shift Arithmetic/1
  Selector6/1 -> Data Type Conversion5/1
  Selector5/1 -> Data Type Conversion4/1
  Data Type Conversion7/1 -> Shift Arithmetic4/1
  Data Type Conversion6/1 -> Add1/1
  Selector7/1 -> Data Type Conversion6/1
  Selector8/1 -> Data Type Conversion7/1
  Data Type Conversion5/1 -> Shift Arithmetic3/1
  In1/1 -> Selector3/1, Selector4/1, Selector2/1, Selector1/1, Selector5/1, Selector6/1, Selector7/1, Selector8/1
  Add1/1 -> Data Type Conversion8/1
  Shift Arithmetic4/1 -> Add1/2
  Data Type Conversion8/1 -> Data Store Write1/1
  Shift Arithmetic3/1 -> Add2/2
  Data Type Conversion4/1 -> Add2/1
  Add2/1 -> Data Type Conversion9/1
  Data Type Conversion9/1 -> Data Store Write3/1

== system DoubleJoints_Algorithm/接收上位机的数据/Subsystem/Joint1 ==
  Joint1 : Inport
  Action Port : ActionPort  ActionType=case
  Data Store Write2 : DataStoreWrite  DataStoreName=J1
  wires:
  Joint1/1 -> Data Store Write2/1

== system DoubleJoints_Algorithm/接收上位机的数据/Subsystem/Joint2 ==
  Joint2 : Inport
  Action Port : ActionPort  ActionType=case
  Data Store Write2 : DataStoreWrite  DataStoreName=J2
  wires:
  Joint2/1 -> Data Store Write2/1

== system DoubleJoints_Algorithm/接收上位机的数据/Subsystem/Joint3 ==
  Joint3 : Inport
  Action Port : ActionPort  ActionType=case
  Data Store Write2 : DataStoreWrite  DataStoreName=J3
  wires:
  Joint3/1 -> Data Store Write2/1

== system DoubleJoints_Algorithm/接收上位机的数据/Subsystem/Joint4 ==
  Joint4 : Inport
  Action Port : ActionPort  ActionType=case
  Data Store Write2 : DataStoreWrite  DataStoreName=J4
  wires:
  Joint4/1 -> Data Store Write2/1

== system DoubleJoints_Algorithm/接收上位机的数据/Subsystem/Joint5 ==
  Joint5 : Inport
  Action Port : ActionPort  ActionType=case
  Data Store Write2 : DataStoreWrite  DataStoreName=J5
  wires:
  Joint5/1 -> Data Store Write2/1

== system DoubleJoints_Algorithm/接收上位机的数据/Subsystem/Joint6 ==
  Joint6 : Inport
  Action Port : ActionPort  ActionType=case
  Data Store Write2 : DataStoreWrite  DataStoreName=J6
  wires:
  Joint6/1 -> Data Store Write2/1

== system DoubleJoints_Algorithm/接收上位机的数据/Subsystem/Joint7 ==
  Joint7 : Inport
  Action Port : ActionPort  ActionType=case
  Data Store Write2 : DataStoreWrite  DataStoreName=J7
  wires:
  Joint7/1 -> Data Store Write2/1

== system DoubleJoints_Algorithm/接收上位机的数据/获取用户命令/消息校验 ==
  数据 : Inport
  Add : Sum  Inputs=8
  Constant : Constant  Value=[0 0 0 0 0 0 0 0 0]  OutDataTypeStr=uint16
  Data Type Conversion : DataTypeConversion  OutDataTypeStr=uint16
  Demux : Demux  Outputs=9
  Relational Operator : RelationalOperator  Operator===  OutDataTypeStr=boolean  RndMeth=Simplest
  Switch : Switch  Criteria=u2 > Threshold
  消息 : Outport
  使能 : Outport  Port=2
  wires:
  数据/1 -> Switch/1, Demux/1
  Demux/1 -> Add/1
  Demux/2 -> Add/2
  Demux/3 -> Add/3
  Demux/4 -> Add/4
  Demux/5 -> Add/5
  Demux/6 -> Add/6
  Demux/7 -> Add/7
  Demux/8 -> Add/8
  Add/1 -> Data Type Conversion/1
  Data Type Conversion/1 -> Relational Operator/1
  Demux/9 -> Relational Operator/2
  Switch/1 -> 消息/1
  Constant/1 -> Switch/3
  Relational Operator/1 -> Switch/2, 使能/1

== system DoubleJoints_Algorithm/DynamicsController/AdapitionController/Controller/Subsystem ==
  note: $s_1$
  note: $\ddot q_{r1}(t)$
  note: $\dot\hat a_1=-\lambda\ddot q_{r1}s_1$
  note: $\hat a_1$
  s1 : Inport
  ddqr_1 : Inport  Port=2
  lambda : Inport  Port=3
  Product : Product
  Product1 : Product
  Product11 : Product
  gain : Gain  Gain=-1
  积分 : Subsystem  TreatAsAtomicUnit=on
  dd_qr1*hat_a1 : Outport
  wires:
  Product1/1 -> gain/1
  积分/1(Out1) -> Product11/2  "hat_a1"
  ddqr_1/1 -> Product11/1, Product1/1
  gain/1 -> Product/1
  Product11/1 -> dd_qr1*hat_a1/1
  s1/1 -> Product1/2
  lambda/1 -> Product/2
  Product/1 -> 积分/1(In1)

== system DoubleJoints_Algorithm/DynamicsController/AdapitionController/Controller/Subsystem1 ==
  note: $\ddot q_{r2}s_1$
  note: $\ddot q_{r1}+\ddot q_{r2}$
  note: $(\ddot q_{r1}+\ddot q_{r2})s_2$
  note: $\dot\hat a_2=-\lambda[\ddot q_{r2}s_1+(\ddot q_{r1}+\ddot q_{r2})s_2]$
  note: $\ddot q_{r2}(t)$
  note: $\hat a_2$
  note: $(\ddot q_{r1}+\ddot q_{r2})\hat a_2$
  note: $\ddot q_{r2}(t)\hat a_2$
  s1 : Inport
  ddqr_1 : Inport  Port=2
  ddqr_2 : Inport  Port=3
  s2 : Inport  Port=4
  lambda : Inport  Port=5
  Add : Sum
  Add3 : Sum
  Product{,2..3,12,17} (5 alike) : Product
  gain : Gain  Gain=-1
  积分 : Subsystem  TreatAsAtomicUnit=on
  ddqr_2*hat_a2 : Outport
  (ddqr_1+ddqr_2)*hat_a2 : Outport  Port=2
  wires:
  Product2/1 -> Add/1
  积分/1(Out1) -> Product12/2, Product17/1
  Product3/1 -> Add/2
  Add3/1 -> Product17/2, Product3/1
  ddqr_2/1 -> Add3/2, Product12/1, Product2/1
  Product/1 -> 积分/1(In1)
  s1/1 -> Product2/2
  Product12/1 -> ddqr_2*hat_a2/1
  Product17/1 -> (ddqr_1+ddqr_2)*hat_a2/1
  s2/1 -> Product3/2
  ddqr_1/1 -> Add3/1
  lambda/1 -> Product/2
  gain/1 -> Product/1
  Add/1 -> gain/1

== system DoubleJoints_Algorithm/DynamicsController/AdapitionController/Controller/Subsystem2 ==
  note: $Y_{13}s_1$
  note: $Y_{23}s_2$
  note: $\dot\hat a_3=-\lambda(Y_{13}s1+Y_{23}s_2)$
  note: $Y_{13}\hat a_3$
  note: $\hat a_3$
  s1 : Inport
  s2 : Inport  Port=2
  Y23 : Inport  Port=3
  Y13 : Inport  Port=4
  lambda : Inport  Port=5
  Add1 : Sum
  Product{,5..6,13} (4 alike) : Product
  gain : Gain  Gain=-1
  积分 : Subsystem  TreatAsAtomicUnit=on
  Y13*hat_a3 : Outport
  hat_a3 : Outport  Port=2
  wires:
  s1/1 -> Product5/1
  积分/1(Out1) -> hat_a3/1, Product13/2
  Product6/1 -> Add1/2
  Y13/1 -> Product13/1, Product5/2
  Product/1 -> 积分/1(In1)
  Product5/1 -> Add1/1
  Y23/1 -> Product6/2
  Product13/1 -> Y13*hat_a3/1
  s2/1 -> Product6/1
  lambda/1 -> Product/2
  gain/1 -> Product/1
  Add1/1 -> gain/1

== system DoubleJoints_Algorithm/DynamicsController/AdapitionController/Controller/Subsystem3 ==
  note: $\dot\hat a_4=-\lambda cos(q_{11})s_1$
  note: $\hat a_4cos(q_{11})$
  s1 : Inport
  q11 : Inport  Port=2
  lambda : Inport  Port=3
  Fcn : Fcn  Expr=cos(u(1))
  Product : Product
  Product14 : Product
  Product7 : Product
  gain : Gain  Gain=-1
  积分 : Subsystem  TreatAsAtomicUnit=on
  cos(q11)*hat_a4 : Outport
  wires:
  s1/1 -> Product7/1
  Fcn/1 -> Product7/2, Product14/2
  Product/1 -> 积分/1(In1)
  Product14/1 -> cos(q11)*hat_a4/1
  q11/1 -> Fcn/1
  积分/1(Out1) -> Product14/1
  lambda/1 -> Product/2
  gain/1 -> Product/1
  Product7/1 -> gain/1

== system DoubleJoints_Algorithm/DynamicsController/AdapitionController/Controller/Subsystem4 ==
  note: $\dot\hat a_5=-\lambda (s_1+s_2)cos(q_{11}+q_{12})$
  note: $\cos(q_{11}+q_{12})\hat a_5$
  s1 : Inport
  s2 : Inport  Port=2
  q11&q12 : Inport  Port=3
  lambda : Inport  Port=4
  Add2 : Sum
  Fcn1 : Fcn  Expr=cos(u(1)+u(2))
  Product : Product
  Product15 : Product
  Product8 : Product
  gain : Gain  Gain=-1
  积分 : Subsystem  TreatAsAtomicUnit=on
  cos(q11+q12)*hat_a5 : Outport
  wires:
  s2/1 -> Add2/2
  Fcn1/1 -> Product15/2, Product8/2
  积分/1(Out1) -> Product15/1
  Add2/1 -> Product8/1
  Product15/1 -> cos(q11+q12)*hat_a5/1
  s1/1 -> Add2/1
  q11&q12/1 -> Fcn1/1
  Product/1 -> 积分/1(In1)
  lambda/1 -> Product/2
  gain/1 -> Product/1
  Product8/1 -> gain/1

== system DoubleJoints_Algorithm/DynamicsController/AdapitionController/Controller/Subsystem5 ==
  note: $\dot f_1=-\lambda \dot q_{r1}s_1$
  note: $\dot q_{r1}\hat f_1$
  s1 : Inport
  dqr_1 : Inport  Port=2
  lambda : Inport  Port=3
  Product : Product
  Product16 : Product
  Product9 : Product
  gain : Gain  Gain=-1
  积分 : Subsystem  TreatAsAtomicUnit=on
  dqr_1*hat_f1 : Outport
  wires:
  s1/1 -> Product9/2
  Product/1 -> 积分/1(In1)
  dqr_1/1 -> Product16/1, Product9/1
  Product16/1 -> dqr_1*hat_f1/1
  积分/1(Out1) -> Product16/2
  lambda/1 -> Product/2
  gain/1 -> Product/1
  Product9/1 -> gain/1

== system DoubleJoints_Algorithm/DynamicsController/AdapitionController/Controller/Subsystem6 ==
  note: $\dot\hat f_2=-\lambda \dot q_{r2}s_2$
  note: $\dot q_{r2}\hat f_2$
  s1 : Inport
  dqr_2 : Inport  Port=2
  lambda : Inport  Port=3
  Product : Product
  Product10 : Product
  Product19 : Product
  gain : Gain  Gain=-1
  积分 : Subsystem  TreatAsAtomicUnit=on
  dqr_2*hat_f2 : Outport
  wires:
  Product/1 -> 积分/1(In1)
  积分/1(Out1) -> Product19/2
  dqr_2/1 -> Product19/1, Product10/1
  Product19/1 -> dqr_2*hat_f2/1
  s1/1 -> Product10/2
  lambda/1 -> Product/2
  gain/1 -> Product/1
  Product10/1 -> gain/1

== system DoubleJoints_Algorithm/DynamicsController/AdapitionController/Controller/Subsystem7 ==
  note: $\pmatrix {q_{11}\cr q_{12}\cr \dot q_{11}\cr \dot q_{12}}$
  ddqr_1 : Inport
  ddqr_2 : Inport  Port=2
  dqr_1 : Inport  Port=3
  q : Inport  Port=4
  dqr_2 : Inport  Port=5
  Demux : Demux
  "Y13 " : Subsystem  TreatAsAtomicUnit=on
  Y23 : Subsystem  TreatAsAtomicUnit=on
  Y13 : Outport
  "Y23 " : Outport  Port=2
  q11 : Outport  Port=3
  wires:
  Demux/3 -> Y23/4(dq11), "Y13 "/6(dq11)
  dqr_1/1 -> Y23/1(dqr1), "Y13 "/1(dqr1)
  "Y13 "/1(Y13) -> Y13/1
  Demux/4 -> "Y13 "/7(dq12)
  Demux/2 -> "Y13 "/5(q12), Y23/3(q12)
  dqr_2/1 -> Y23/2(ddqr1), "Y13 "/2(dqr2)
  ddqr_1/1 -> "Y13 "/3(ddqr1)
  ddqr_2/1 -> "Y13 "/4(ddqr2)
  Y23/1(Y23) -> "Y23 "/1
  q/1 -> Demux/1
  Demux/1 -> q11/1

== system DoubleJoints_Algorithm/DynamicsController/AdapitionController/Error /Subsystem ==
  note: $e_{11}(t)=q_{11}(t)-q_{d1}(t)$
  q11 : Inport
  gain : Inport  Port=2
  Enable : EnablePort
  Product : Product
  Sum : Sum  Inputs=|+-
  ref_signal : dspsrcs4/Sine Wave  Amplitude=1  Frequency=Freq  Phase=0  SampleMode=Discrete  OutComplex=Real  CompMethod=Trigonometric fcn  TableSize=Speed  SampleTime=SimpleTime  SamplesPerFrame=1  ResetState=Restart at time zero  OutputFrames=on  dataType=double  wordLen=16  udDataType=sfix(16)  fracBitsMode=Best precision  numFracBits=15  OutDataTypeStr=double  LastOutDataTypeStr=double
  e11 : Outport
  qd1 : Outport  Port=2
  wires:
  ref_signal/1 -> Product/1
  Product/1 -> Sum/2, qd1/1
  gain/1 -> Product/2
  q11/1 -> Sum/1
  Sum/1 -> e11/1

== system DoubleJoints_Algorithm/DynamicsController/AdapitionController/Error /Subsystem1 ==
  note: $e_{12}(t)=q_{12}(t)-q_{d2}(t)$
  q12 : Inport
  gain : Inport  Port=2
  Enable : EnablePort
  Product : Product
  Sum5 : Sum  Inputs=|+-
  ref_signal : dspsrcs4/Sine Wave  Amplitude=1  Frequency=Freq  Phase=0  SampleMode=Discrete  OutComplex=Real  CompMethod=Trigonometric fcn  TableSize=Speed  SampleTime=SimpleTime  SamplesPerFrame=1  ResetState=Restart at time zero  OutputFrames=on  dataType=double  wordLen=16  udDataType=sfix(16)  fracBitsMode=Best precision  numFracBits=15  OutDataTypeStr=double  LastOutDataTypeStr=double
  e12 : Outport
  qd2 : Outport  Port=2
  wires:
  Product/1 -> Sum5/2, qd2/1
  ref_signal/1 -> Product/1
  gain/1 -> Product/2
  Sum5/1 -> e12/1
  q12/1 -> Sum5/1

== system DoubleJoints_Algorithm/DynamicsController/DriverTwoMotor/BottomDriver/Judgement ==
  note: CAN mbx=7
  note: CAN mbx=8
  SelectJointOne : Inport
  SelectJointTwo : Inport  Port=2
  MSG1 : Inport  Port=3
  MSG2 : Inport  Port=4
  Enable : EnablePort
  Constant : Constant  Value=0  OutDataTypeStr=uint8
  Data Store Write : DataStoreWrite  DataStoreName=TWO_TXD
  OneJoint : Subsystem  Priority=1  TreatAsAtomicUnit=on
      settings: RTWSystemCode=Nonreusable function
  TwoJoint : Subsystem  Priority=2  TreatAsAtomicUnit=on
      settings: RTWSystemCode=Nonreusable function
  wires:
  SelectJointOne/1 -> OneJoint/1(In1)
  MSG1/1 -> OneJoint/2(MSG1)
  SelectJointTwo/1 -> TwoJoint/1(In2)
  MSG2/1 -> TwoJoint/2(MSG2)
  Constant/1 -> Data Store Write/1

== system DoubleJoints_Algorithm/DynamicsController/DriverTwoMotor/驱动器指令/Chart2/BG ==
  note: 位
      | 置
  note: 电流
  note: 命令
  f : TriggerPort  TriggerType=function-call  VariantControl=(inherit)
      settings: CopyFcn=Stateflow.SLINSF.SimulinkMan.removeBlockPreDeleteFcn  PreDeleteFcn=Stateflow.SLINSF.SimulinkMan.unsafePredeleteFcn
  Constant1 : Constant  Value=hex2dec('47')  OutDataTypeStr=uint8
  Constant2 : Constant  Value=0  VectorParams1D=off  OutDataTypeStr=uint8  SampleTime=-1
  Constant3 : Constant  Value=0  VectorParams1D=off  OutDataTypeStr=uint8  SampleTime=-1
  Constant6 : Constant  OutDataTypeStr=uint8
  Constant8 : Constant  Value=hex2dec('42')  OutDataTypeStr=uint8
  Data Store Write : DataStoreWrite  DataStoreName=TWO_TXD
  Data Type Conversion : DataTypeConversion  OutDataTypeStr=uint16
  Data Type Conversion{1..6} (6 alike) : DataTypeConversion  OutDataTypeStr=uint8
  Mux3 : Mux  Inputs=8
  Shift Arithmetic1 : ArithShift  BitShiftNumber=8  BitShiftDirection=Right
  Shift Arithmetic2 : ArithShift  BitShiftNumber=16  BitShiftDirection=Right
  Shift Arithmetic3 : ArithShift  BitShiftNumber=24  BitShiftDirection=Right
  Shift Arithmetic4 : ArithShift  BitShiftNumber=8  BitShiftDirection=Right
  MSG1 : Outport  OutDataTypeStr=uint16  PortDimensions=8
  MSG2 : Outport  Port=2  OutDataTypeStr=uint16  PortDimensions=8
  wires:
  Shift Arithmetic1/1 -> Data Type Conversion3/1
  Shift Arithmetic4/1 -> Data Type Conversion6/1
  Shift Arithmetic3/1 -> Data Type Conversion5/1
  Constant2/1 -> Data Type Conversion1/1, Shift Arithmetic4/1
  Data Type Conversion1/1 -> Mux3/3
  Shift Arithmetic2/1 -> Data Type Conversion4/1
  Data Type Conversion3/1 -> Mux3/6
  Data Type Conversion6/1 -> Mux3/4
  Constant8/1 -> Mux3/1
  Constant1/1 -> Mux3/2
  Data Type Conversion4/1 -> Mux3/7
  Data Type Conversion5/1 -> Mux3/8
  Constant3/1 -> Shift Arithmetic3/1, Shift Arithmetic2/1, Shift Arithmetic1/1, Data Type Conversion2/1
  Data Type Conversion2/1 -> Mux3/5
  Constant6/1 -> Data Store Write/1
  Data Type Conversion/1 -> MSG1/1, MSG2/1
  Mux3/1 -> Data Type Conversion/1

== system DoubleJoints_Algorithm/DynamicsController/DriverTwoMotor/驱动器指令/Chart2/TF ==
  Current1 : Inport  OutDataTypeStr=uint16  PortDimensions=1
  Current2 : Inport  Port=2  OutDataTypeStr=uint16  PortDimensions=1
  f : TriggerPort  TriggerType=function-call  VariantControl=(inherit)
      settings: CopyFcn=Stateflow.SLINSF.SimulinkMan.removeBlockPreDeleteFcn  PreDeleteFcn=Stateflow.SLINSF.SimulinkMan.unsafePredeleteFcn
  Constant2 : Constant  OutDataTypeStr=uint8
  Data Store Write : DataStoreWrite  DataStoreName=TWO_TXD
  TF : Subsystem  TreatAsAtomicUnit=on
  TF1 : Subsystem  TreatAsAtomicUnit=on
  MSG1 : Outport  OutDataTypeStr=uint16  PortDimensions=8
  MSG2 : Outport  Port=2  OutDataTypeStr=uint16  PortDimensions=8
  wires:
  Constant2/1 -> Data Store Write/1
  TF1/1(MSG) -> MSG2/1
  Current1/1 -> TF/1(Current)
  TF/1(MSG) -> MSG1/1
  Current2/1 -> TF1/1(Current)

== system DoubleJoints_Algorithm/DynamicsController/DriverTwoMotor/驱动器指令/Chart2/UM1 ==
  note: 电流
  note: 位
      | 置
  note: 命令
  f : TriggerPort  TriggerType=function-call  VariantControl=(inherit)
      settings: CopyFcn=Stateflow.SLINSF.SimulinkMan.removeBlockPreDeleteFcn  PreDeleteFcn=Stateflow.SLINSF.SimulinkMan.unsafePredeleteFcn
  Constant : Constant  OutDataTypeStr=uint8
  Constant1 : Constant  Value=hex2dec('4d')  OutDataTypeStr=uint8
  Constant2 : Constant  Value=0  VectorParams1D=off  OutDataTypeStr=uint8  SampleTime=-1
  Constant3 : Constant  VectorParams1D=off  OutDataTypeStr=uint8  SampleTime=-1
  Constant8 : Constant  Value=hex2dec('55')  OutDataTypeStr=uint8
  Data Store Write : DataStoreWrite  DataStoreName=TWO_TXD
  Data Type Conversion : DataTypeConversion  OutDataTypeStr=uint16
  Data Type Conversion{1..6} (6 alike) : DataTypeConversion  OutDataTypeStr=uint8
  Mux3 : Mux  Inputs=8
  Shift Arithmetic1 : ArithShift  BitShiftNumber=8  BitShiftDirection=Right
  Shift Arithmetic2 : ArithShift  BitShiftNumber=16  BitShiftDirection=Right
  Shift Arithmetic3 : ArithShift  BitShiftNumber=24  BitShiftDirection=Right
  Shift Arithmetic4 : ArithShift  BitShiftNumber=8  BitShiftDirection=Right
  MSG1 : Outport  OutDataTypeStr=uint16  PortDimensions=8
  MSG2 : Outport  Port=2  OutDataTypeStr=uint16  PortDimensions=8
  wires:
  Constant/1 -> Data Store Write/1
  Data Type Conversion4/1 -> Mux3/7
  Shift Arithmetic2/1 -> Data Type Conversion4/1
  Data Type Conversion1/1 -> Mux3/3
  Shift Arithmetic4/1 -> Data Type Conversion6/1
  Data Type Conversion3/1 -> Mux3/6
  Data Type Conversion6/1 -> Mux3/4
  Data Type Conversion5/1 -> Mux3/8
  Shift Arithmetic3/1 -> Data Type Conversion5/1
  Constant1/1 -> Mux3/2
  Shift Arithmetic1/1 -> Data Type Conversion3/1
  Constant3/1 -> Shift Arithmetic1/1, Data Type Conversion2/1, Shift Arithmetic2/1, Shift Arithmetic3/1
  Data Type Conversion2/1 -> Mux3/5
  Constant2/1 -> Shift Arithmetic4/1, Data Type Conversion1/1
  Constant8/1 -> Mux3/1
  Data Type Conversion/1 -> MSG2/1, MSG1/1
  Mux3/1 -> Data Type Conversion/1

== system DoubleJoints_Algorithm/DynamicsController/DriverTwoMotor/驱动器指令/Chart2/check ==
  write : Inport  OutDataTypeStr=uint16  PortDimensions=1
  f : TriggerPort  TriggerType=function-call  VariantControl=(inherit)
      settings: CopyFcn=Stateflow.SLINSF.SimulinkMan.removeBlockPreDeleteFcn  PreDeleteFcn=Stateflow.SLINSF.SimulinkMan.unsafePredeleteFcn
  Constant : Constant  OutDataTypeStr=uint16
  Constant1 : Constant  Value=0  OutDataTypeStr=uint16
  Data Type Conversion : DataTypeConversion  OutDataTypeStr=uint16
  Switch : Switch  Criteria=u2 > Threshold  OutDataTypeStr=uint16
  bx : Outport  OutDataTypeStr=uint16  PortDimensions=1
  wires:
  Switch/1 -> Data Type Conversion/1
  Constant1/1 -> Switch/3
  Constant/1 -> Switch/1
  write/1 -> Switch/2
  Data Type Conversion/1 -> bx/1

== system DoubleJoints_Algorithm/DynamicsController/DriverTwoMotor/驱动器指令/Chart2/start_arm ==
  StartRobot : Inport  OutDataTypeStr=uint16  PortDimensions=1
  f : TriggerPort  TriggerType=function-call  VariantControl=(inherit)
      settings: CopyFcn=Stateflow.SLINSF.SimulinkMan.removeBlockPreDeleteFcn  PreDeleteFcn=Stateflow.SLINSF.SimulinkMan.unsafePredeleteFcn
  Constant : Constant  OutDataTypeStr=uint16
  StartRobotSubsystem : Subsystem
      settings: RTWSystemCode=Nonreusable function
  start : Outport  OutDataTypeStr=uint16  PortDimensions=1
  wires:
  StartRobot/1 -> StartRobotSubsystem/Enable
  StartRobotSubsystem/1(Out1) -> start/1
  Constant/1 -> StartRobotSubsystem/1(In1)

== system DoubleJoints_Algorithm/DynamicsController/AdapitionController/Controller/Subsystem/积分 ==
  In1 : Inport
  Add1 : Sum  Inputs=3
  Add5 : Sum  Inputs=+-
  Delay2 : Delay  DelayLength=1  InitialCondition=0  UseCircularBuffer=on
  Delay3 : Delay  DelayLength=1  InitialCondition=0  UseCircularBuffer=on
  Kc2 : Constant  Value=0.002  OutDataTypeStr=fixdt(1,32,17)
  Product1 : Product
  Saturation2 : Saturate  UpperLimit=1000  LowerLimit=-1000
  Out1 : Outport
  wires:
  Delay3/1 -> Product1/1
  Delay2/1 -> Add1/1
  Add1/1 -> Delay2/1, Add5/2, Saturation2/1
  Product1/1 -> Add1/3
  Add5/1 -> Delay3/1
  Saturation2/1 -> Add5/1, Out1/1
  Kc2/1 -> Product1/2
  In1/1 -> Add1/2
